simulink model "sscv_braking_ABS_w_vehicle"  (R2024a)
settings: Solver=ode23t  StartTime=0.0  StopTime=1  RelTol=1e-3  AbsTol=1e-3
PreLoadFcn:
  | sscv_braking_ABS_w_vehicle_input
values from neighbouring files (symbols this model uses):
  wheel_rad = 0.3    [sscv_braking_ABS_w_vehicle_input.m]
  wheel_vth = 0.01    [sscv_braking_ABS_w_vehicle_input.m]
undefined symbols (not defined in the file or in its folder): Asphalt, fcdb, HCU, MFormulaCoeff, tpc, vb
libraries: fl_lib x165, SimscapeFluids_lib x24, nesl_utility x21, sdl_lib x9, simulink x3, simulink_extras x1
(part 2 of 6)

== system sscv_braking_ABS_w_vehicle/Brakes with ABS/FCDB/RLW ==
  CP1 : fl_lib/Isothermal Liquid/Elements/Translational Mechanical Converter (IL)  mech_orientation=1  displacement_spec=foundation.enum.DisplacementSpec.Calculate  x0=0 m  interface_area=fcdb.area m^2  dead_volume=fcdb.deadV m^3  pressure_spec=1  environment_pressure=0.101325 MPa  dynamic_compressibility=simscape.enum.onoff.on  p0=tpc.pRes Pa
      settings: InternalSimscapePortConfiguration="{\"Bottom\":[],\"Left\":[{\"id\":\"A\",\"label\":\"A\",\"type\":\"foundation.isothermal_liquid.isothermal_liquid\"},{\"id\":\"C\",\"label\":\"C\",\"type\":\"foundation.mechanical.translational.translational\"}],\"Right\":[{\"id\":\"R\",\"label\":\"R\",\"type\":\"foundation.mechanical.translational.translational\"}],\"Top\":[]}"
  CP2 : fl_lib/Isothermal Liquid/Elements/Translational Mechanical Converter (IL)  mech_orientation=1  displacement_spec=foundation.enum.DisplacementSpec.Calculate  x0=0 m  interface_area=fcdb.area m^2  dead_volume=fcdb.deadV m^3  pressure_spec=1  environment_pressure=0.101325 MPa  dynamic_compressibility=simscape.enum.onoff.on  p0=tpc.pRes Pa
      settings: InternalSimscapePortConfiguration="{\"Bottom\":[],\"Left\":[{\"id\":\"A\",\"label\":\"A\",\"type\":\"foundation.isothermal_liquid.isothermal_liquid\"},{\"id\":\"C\",\"label\":\"C\",\"type\":\"foundation.mechanical.translational.translational\"}],\"Right\":[{\"id\":\"R\",\"label\":\"R\",\"type\":\"foundation.mechanical.translational.translational\"}],\"Top\":[]}"
  Ideal Force Sensor : fl_lib/Mechanical/Mechanical Sensors/Ideal Force Sensor
  Ideal Force Sensor1 : fl_lib/Mechanical/Mechanical Sensors/Ideal Force Sensor
  Loaded-Contact Rotational Friction : sdl_lib/Brakes & Detents/Rotational/Loaded-Contact Rotational Friction  geometry_model=sdl.enum.friction_geometry.radius  r_eff=fcdb.reffR m  d_o=150 mm  d_i=100 mm  enable_faults=simscape.enum.onoff.off  fault_type=sdl.enum.clutchFault.lock  friction_model=sdl.enum.friction_model_TLU_thermal.fixed  mu_w_vector=[0, 100, 1000] rad/s  temperature_TLU=[280, 300, 320] K  mu_static=fcdb.statFric  mu_static_vector=[.4, .38, .36]  mu_coulomb=fcdb.kinFric  mu_coulomb_vector=[.3, .22, .19]  mu_coulomb_temp_vector=[.3, .28, .25]  mu_coulomb_matrix=[.34, .32, .3; .3, .28, .25; .25, .2, .15]  mu_interp_method=simscape.enum.interpolation.linear  mu_extrap_method=simscape.enum.extrapolation.linear  w_tol=0.01 rad/s  force_min=1 N  mu_visc=fcdb.dampDisk N*m/(rad/s)  initial_state_locked=sdl.enum.initial_lock.unlocked  thermal_mass=50 kJ/K  T_init=300 K
      settings: InternalSimscapePortConfiguration="{\"Bottom\":[],\"Left\":[{\"id\":\"N\",\"label\":\"N\",\"type\":\"input\"},{\"id\":\"B\",\"label\":\"B\",\"type\":\"foundation.mechanical.rotational.rotational\"}],\"Right\":[{\"id\":\"F\",\"label\":\"F\",\"type\":\"foundation.mechanical.rotational.rotational\"}],\"Top\":[]}"
  Mass : fl_lib/Mechanical/Translational Elements/Mass  mass=fcdb.mass kg  num_ports=foundation.enum.numPorts2.one  v_specify=off  v_priority=High  v=0 m/s  v_nominal_specify=off  v_nominal_value=1  v_nominal_unit=m/s  f_specify=off  f_priority=None  f=0 N  f_nominal_specify=off  f_nominal_value=1  f_nominal_unit=N
  Mass1 : fl_lib/Mechanical/Translational Elements/Mass  mass=fcdb.mass kg  num_ports=foundation.enum.numPorts2.one  v_specify=off  v_priority=High  v=0 m/s  v_nominal_specify=off  v_nominal_value=1  v_nominal_unit=m/s  f_specify=off  f_priority=None  f=0 N  f_nominal_specify=off  f_nominal_value=1  f_nominal_unit=N
  Mechanical Rotational Reference : fl_lib/Mechanical/Rotational Elements/Mechanical Rotational Reference
  Mechanical Translational Reference : fl_lib/Mechanical/Translational Elements/Mechanical Translational Reference
  PS Add : fl_lib/Physical Signals/Functions/PS Add
  Translational Damper : fl_lib/Mechanical/Translational Elements/Translational Damper  D=fcdb.damp N/(m/s)  v_specify=off  v_priority=None  v=0 m/s  v_nominal_specify=off  v_nominal_value=1  v_nominal_unit=m/s  f_specify=off  f_priority=None  f=0 N  f_nominal_specify=off  f_nominal_value=1  f_nominal_unit=N
  Translational Damper1 : fl_lib/Mechanical/Translational Elements/Translational Damper  D=fcdb.damp N/(m/s)  v_specify=off  v_priority=None  v=0 m/s  v_nominal_specify=off  v_nominal_value=1  v_nominal_unit=m/s  f_specify=off  f_priority=None  f=0 N  f_nominal_specify=off  f_nominal_value=1  f_nominal_unit=N
  Translational Hard Stop : fl_lib/Mechanical/Translational Elements/Translational Hard Stop  upper_bnd=fcdb.runClear m  lower_bnd=0 m  model=simscape.enum.hardstop.smooth  stiff_up=fcdb.complianceR N/m  stiff_low=fcdb.hss N/m  D_up=fcdb.damp N/(m/s)  D_low=fcdb.hsd N/(m/s)  transition=0.1 mm  coeff_rest=0.7  v_tol=0.001 m/s  f_tol=0.001 N  v_specify=off  v_priority=None  v=0 m/s  v_nominal_specify=off  v_nominal_value=1  v_nominal_unit=m/s  f_specify=off  f_priority=None  f=0 N  f_nominal_specify=off  f_nominal_value=1  f_nominal_unit=N  x_specify=off  x_priority=High  x=0 m  x_nominal_specify=off  x_nominal_value=1  x_nominal_unit=m  M_specify=off  M_priority=None  M=0
  Translational Hard Stop1 : fl_lib/Mechanical/Translational Elements/Translational Hard Stop  upper_bnd=fcdb.runClear m  lower_bnd=0 m  model=simscape.enum.hardstop.smooth  stiff_up=fcdb.complianceR N/m  stiff_low=fcdb.hss N/m  D_up=fcdb.damp N/(m/s)  D_low=fcdb.hsd N/(m/s)  transition=0.1 mm  coeff_rest=0.7  v_tol=0.001 m/s  f_tol=0.001 N  v_specify=off  v_priority=None  v=0 m/s  v_nominal_specify=off  v_nominal_value=1  v_nominal_unit=m/s  f_specify=off  f_priority=None  f=0 N  f_nominal_specify=off  f_nominal_value=1  f_nominal_unit=N  x_specify=off  x_priority=High  x=0 m  x_nominal_specify=off  x_nominal_value=1  x_nominal_unit=m  M_specify=off  M_priority=None  M=0
  Brk2 : PMIOPort  Side=Left
  TRLW : PMIOPort  Port=2  Side=Right
  connections:
  Ideal Force Sensor/LConn1 -- Translational Damper/RConn1 -- Translational Hard Stop/RConn1
  Ideal Force Sensor/RConn1 -- CP1/LConn2 -- CP2/LConn2 -- Ideal Force Sensor1/RConn1 -- Mechanical Translational Reference/LConn1
  Translational Damper1/LConn1 -- CP2/RConn1 -- Mass1/LConn1 -- Translational Hard Stop1/LConn1
  Ideal Force Sensor1/LConn1 -- Translational Damper1/RConn1 -- Translational Hard Stop1/RConn1
  PS Add/LConn1 -- Ideal Force Sensor/RConn2
  Ideal Force Sensor1/RConn2 -- PS Add/LConn2
  PS Add/RConn1 -- Loaded-Contact Rotational Friction/LConn1
  Mechanical Rotational Reference/LConn1 -- Loaded-Contact Rotational Friction/LConn2
  TRLW/RConn1 -- Loaded-Contact Rotational Friction/RConn1
  Brk2/RConn1 -- CP2/LConn1 -- CP1/LConn1
  Translational Damper/LConn1 -- Mass/LConn1 -- CP1/RConn1 -- Translational Hard Stop/LConn1

== system sscv_braking_ABS_w_vehicle/Brakes with ABS/FCDB/RRW ==
  CP1 : fl_lib/Isothermal Liquid/Elements/Translational Mechanical Converter (IL)  mech_orientation=1  displacement_spec=foundation.enum.DisplacementSpec.Calculate  x0=0 m  interface_area=fcdb.area m^2  dead_volume=fcdb.deadV m^3  pressure_spec=1  environment_pressure=0.101325 MPa  dynamic_compressibility=simscape.enum.onoff.on  p0=tpc.pRes Pa
      settings: InternalSimscapePortConfiguration="{\"Bottom\":[],\"Left\":[{\"id\":\"A\",\"label\":\"A\",\"type\":\"foundation.isothermal_liquid.isothermal_liquid\"},{\"id\":\"C\",\"label\":\"C\",\"type\":\"foundation.mechanical.translational.translational\"}],\"Right\":[{\"id\":\"R\",\"label\":\"R\",\"type\":\"foundation.mechanical.translational.translational\"}],\"Top\":[]}"
  CP2 : fl_lib/Isothermal Liquid/Elements/Translational Mechanical Converter (IL)  mech_orientation=1  displacement_spec=foundation.enum.DisplacementSpec.Calculate  x0=0 m  interface_area=fcdb.area m^2  dead_volume=fcdb.deadV m^3  pressure_spec=1  environment_pressure=0.101325 MPa  dynamic_compressibility=simscape.enum.onoff.on  p0=tpc.pRes Pa
      settings: InternalSimscapePortConfiguration="{\"Bottom\":[],\"Left\":[{\"id\":\"A\",\"label\":\"A\",\"type\":\"foundation.isothermal_liquid.isothermal_liquid\"},{\"id\":\"C\",\"label\":\"C\",\"type\":\"foundation.mechanical.translational.translational\"}],\"Right\":[{\"id\":\"R\",\"label\":\"R\",\"type\":\"foundation.mechanical.translational.translational\"}],\"Top\":[]}"
  Ideal Force Sensor : fl_lib/Mechanical/Mechanical Sensors/Ideal Force Sensor
  Ideal Force Sensor1 : fl_lib/Mechanical/Mechanical Sensors/Ideal Force Sensor
  Loaded-Contact Rotational Friction : sdl_lib/Brakes & Detents/Rotational/Loaded-Contact Rotational Friction  geometry_model=sdl.enum.friction_geometry.radius  r_eff=fcdb.reffR m  d_o=150 mm  d_i=100 mm  enable_faults=simscape.enum.onoff.off  fault_type=sdl.enum.clutchFault.lock  friction_model=sdl.enum.friction_model_TLU_thermal.fixed  mu_w_vector=[0, 100, 1000] rad/s  temperature_TLU=[280, 300, 320] K  mu_static=fcdb.statFric  mu_static_vector=[.4, .38, .36]  mu_coulomb=fcdb.kinFric  mu_coulomb_vector=[.3, .22, .19]  mu_coulomb_temp_vector=[.3, .28, .25]  mu_coulomb_matrix=[.34, .32, .3; .3, .28, .25; .25, .2, .15]  mu_interp_method=simscape.enum.interpolation.linear  mu_extrap_method=simscape.enum.extrapolation.linear  w_tol=0.01 rad/s  force_min=1 N  mu_visc=fcdb.dampDisk N*m/(rad/s)  initial_state_locked=sdl.enum.initial_lock.unlocked  thermal_mass=50 kJ/K  T_init=300 K
      settings: InternalSimscapePortConfiguration="{\"Bottom\":[],\"Left\":[{\"id\":\"N\",\"label\":\"N\",\"type\":\"input\"},{\"id\":\"B\",\"label\":\"B\",\"type\":\"foundation.mechanical.rotational.rotational\"}],\"Right\":[{\"id\":\"F\",\"label\":\"F\",\"type\":\"foundation.mechanical.rotational.rotational\"}],\"Top\":[]}"
  Mass : fl_lib/Mechanical/Translational Elements/Mass  mass=fcdb.mass kg  num_ports=foundation.enum.numPorts2.one  v_specify=off  v_priority=High  v=0 m/s  v_nominal_specify=off  v_nominal_value=1  v_nominal_unit=m/s  f_specify=off  f_priority=None  f=0 N  f_nominal_specify=off  f_nominal_value=1  f_nominal_unit=N
  Mass1 : fl_lib/Mechanical/Translational Elements/Mass  mass=fcdb.mass kg  num_ports=foundation.enum.numPorts2.one  v_specify=off  v_priority=High  v=0 m/s  v_nominal_specify=off  v_nominal_value=1  v_nominal_unit=m/s  f_specify=off  f_priority=None  f=0 N  f_nominal_specify=off  f_nominal_value=1  f_nominal_unit=N
  Mechanical Rotational Reference : fl_lib/Mechanical/Rotational Elements/Mechanical Rotational Reference
  Mechanical Translational Reference : fl_lib/Mechanical/Translational Elements/Mechanical Translational Reference
  PS Add : fl_lib/Physical Signals/Functions/PS Add
  Translational Damper : fl_lib/Mechanical/Translational Elements/Translational Damper  D=fcdb.damp N/(m/s)  v_specify=off  v_priority=None  v=0 m/s  v_nominal_specify=off  v_nominal_value=1  v_nominal_unit=m/s  f_specify=off  f_priority=None  f=0 N  f_nominal_specify=off  f_nominal_value=1  f_nominal_unit=N
  Translational Damper1 : fl_lib/Mechanical/Translational Elements/Translational Damper  D=fcdb.damp N/(m/s)  v_specify=off  v_priority=None  v=0 m/s  v_nominal_specify=off  v_nominal_value=1  v_nominal_unit=m/s  f_specify=off  f_priority=None  f=0 N  f_nominal_specify=off  f_nominal_value=1  f_nominal_unit=N
  Translational Hard Stop : fl_lib/Mechanical/Translational Elements/Translational Hard Stop  upper_bnd=fcdb.runClear m  lower_bnd=0 m  model=simscape.enum.hardstop.smooth  stiff_up=fcdb.complianceR N/m  stiff_low=fcdb.hss N/m  D_up=fcdb.damp N/(m/s)  D_low=fcdb.hsd N/(m/s)  transition=0.1 mm  coeff_rest=0.7  v_tol=0.001 m/s  f_tol=0.001 N  v_specify=off  v_priority=None  v=0 m/s  v_nominal_specify=off  v_nominal_value=1  v_nominal_unit=m/s  f_specify=off  f_priority=None  f=0 N  f_nominal_specify=off  f_nominal_value=1  f_nominal_unit=N  x_specify=off  x_priority=High  x=0 m  x_nominal_specify=off  x_nominal_value=1  x_nominal_unit=m  M_specify=off  M_priority=None  M=0
  Translational Hard Stop1 : fl_lib/Mechanical/Translational Elements/Translational Hard Stop  upper_bnd=fcdb.runClear m  lower_bnd=0 m  model=simscape.enum.hardstop.smooth  stiff_up=fcdb.complianceR N/m  stiff_low=fcdb.hss N/m  D_up=fcdb.damp N/(m/s)  D_low=fcdb.hsd N/(m/s)  transition=0.1 mm  coeff_rest=0.7  v_tol=0.001 m/s  f_tol=0.001 N  v_specify=off  v_priority=None  v=0 m/s  v_nominal_specify=off  v_nominal_value=1  v_nominal_unit=m/s  f_specify=off  f_priority=None  f=0 N  f_nominal_specify=off  f_nominal_value=1  f_nominal_unit=N  x_specify=off  x_priority=High  x=0 m  x_nominal_specify=off  x_nominal_value=1  x_nominal_unit=m  M_specify=off  M_priority=None  M=0
  Brk2 : PMIOPort  Side=Left
  TRRW : PMIOPort  Port=2  Side=Right
  connections:
  Ideal Force Sensor1/RConn2 -- PS Add/LConn2
  PS Add/LConn1 -- Ideal Force Sensor/RConn2
  Translational Damper1/RConn1 -- Translational Hard Stop1/RConn1 -- Ideal Force Sensor1/LConn1
  Mechanical Translational Reference/LConn1 -- Ideal Force Sensor1/RConn1 -- CP2/LConn2 -- Ideal Force Sensor/RConn1 -- CP1/LConn2
  Translational Hard Stop/RConn1 -- Translational Damper/RConn1 -- Ideal Force Sensor/LConn1
  PS Add/RConn1 -- Loaded-Contact Rotational Friction/LConn1
  Mechanical Rotational Reference/LConn1 -- Loaded-Contact Rotational Friction/LConn2
  TRRW/RConn1 -- Loaded-Contact Rotational Friction/RConn1
  Mass/LConn1 -- Translational Hard Stop/LConn1 -- Translational Damper/LConn1 -- CP1/RConn1
  Brk2/RConn1 -- CP2/LConn1 -- CP1/LConn1
  Translational Hard Stop1/LConn1 -- Mass1/LConn1 -- CP2/RConn1 -- Translational Damper1/LConn1

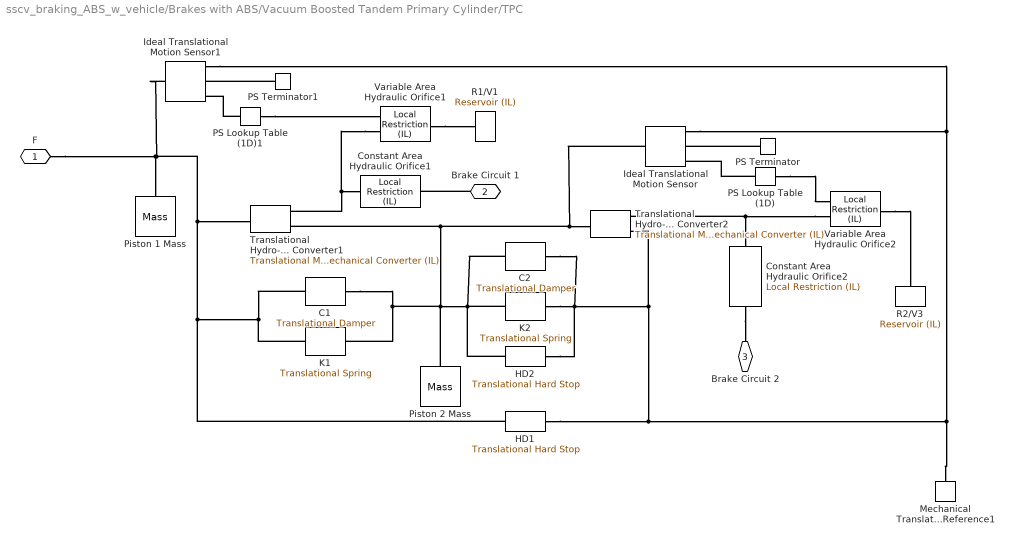
== system sscv_braking_ABS_w_vehicle/Brakes with ABS/Vacuum Boosted Tandem Primary Cylinder/TPC ==
  C1 : fl_lib/Mechanical/Translational Elements/Translational Damper  D=tpc.c1 N/(m/s)  v_specify=off  v_priority=None  v=0 m/s  v_nominal_specify=off  v_nominal_value=1  v_nominal_unit=m/s  f_specify=off  f_priority=None  f=0 N  f_nominal_specify=off  f_nominal_value=1  f_nominal_unit=N
  C2 : fl_lib/Mechanical/Translational Elements/Translational Damper  D=tpc.c2 N/(m/s)  v_specify=off  v_priority=None  v=0 m/s  v_nominal_specify=off  v_nominal_value=1  v_nominal_unit=m/s  f_specify=off  f_priority=None  f=0 N  f_nominal_specify=off  f_nominal_value=1  f_nominal_unit=N
  Constant Area Hydraulic Orifice1 : fl_lib/Isothermal Liquid/Elements/Local Restriction (IL)  restriction_type=1  restriction_area=tpc.a2Ori m^2  min_area=1e-10 m^2  max_area=0.005 m^2  area=inf m^2  Cd=0.7  Re_c=150  pressure_recovery=simscape.enum.onoff.off
      settings: InternalSimscapePortConfiguration="{\"Bottom\":[],\"Left\":[{\"id\":\"A\",\"label\":\"A\",\"type\":\"foundation.isothermal_liquid.isothermal_liquid\"}],\"Right\":[{\"id\":\"B\",\"label\":\"B\",\"type\":\"foundation.isothermal_liquid.isothermal_liquid\"}],\"Top\":[]}"
  Constant Area Hydraulic Orifice2 : fl_lib/Isothermal Liquid/Elements/Local Restriction (IL)  restriction_type=1  restriction_area=tpc.a2Ori m^2  min_area=1e-10 m^2  max_area=0.005 m^2  area=inf m^2  Cd=0.7  Re_c=150  pressure_recovery=simscape.enum.onoff.off
      settings: InternalSimscapePortConfiguration="{\"Bottom\":[],\"Left\":[{\"id\":\"A\",\"label\":\"A\",\"type\":\"foundation.isothermal_liquid.isothermal_liquid\"}],\"Right\":[{\"id\":\"B\",\"label\":\"B\",\"type\":\"foundation.isothermal_liquid.isothermal_liquid\"}],\"Top\":[]}"
  HD1 : fl_lib/Mechanical/Translational Elements/Translational Hard Stop  upper_bnd=tpc.x13 m  lower_bnd=0 m  model=simscape.enum.hardstop.smooth  stiff_up=tpc.hss N/m  stiff_low=tpc.hss N/m  D_up=tpc.hsd N/(m/s)  D_low=tpc.hsd N/(m/s)  transition=0.1 mm  coeff_rest=0.7  v_tol=0.001 m/s  f_tol=0.001 N  v_specify=off  v_priority=None  v=0 m/s  v_nominal_specify=off  v_nominal_value=1  v_nominal_unit=m/s  f_specify=off  f_priority=None  f=0 N  f_nominal_specify=off  f_nominal_value=1  f_nominal_unit=N  x_specify=off  x_priority=High  x=0 m  x_nominal_specify=off  x_nominal_value=1  x_nominal_unit=m  M_specify=off  M_priority=None  M=0
  HD2 : fl_lib/Mechanical/Translational Elements/Translational Hard Stop  upper_bnd=tpc.x23 m  lower_bnd=0 m  model=simscape.enum.hardstop.smooth  stiff_up=tpc.hss N/m  stiff_low=tpc.hss N/m  D_up=tpc.hsd N/(m/s)  D_low=tpc.hsd N/(m/s)  transition=0.1 mm  coeff_rest=0.7  v_tol=0.001 m/s  f_tol=0.001 N  v_specify=off  v_priority=None  v=0 m/s  v_nominal_specify=off  v_nominal_value=1  v_nominal_unit=m/s  f_specify=off  f_priority=None  f=0 N  f_nominal_specify=off  f_nominal_value=1  f_nominal_unit=N  x_specify=off  x_priority=High  x=0 m  x_nominal_specify=off  x_nominal_value=1  x_nominal_unit=m  M_specify=off  M_priority=None  M=0
  Ideal Translational Motion Sensor : fl_lib/Mechanical/Mechanical Sensors/Ideal Translational Motion Sensor  reference=foundation.enum.MeasurementReference.difference  acceleration_port=false  velocity_port=true  position_port=true  offset=0 m
  Ideal Translational Motion Sensor1 : fl_lib/Mechanical/Mechanical Sensors/Ideal Translational Motion Sensor  reference=foundation.enum.MeasurementReference.difference  acceleration_port=false  velocity_port=true  position_port=true  offset=0 m
  K1 : fl_lib/Mechanical/Translational Elements/Translational Spring  spr_rate=tpc.k1 N/m  v_specify=off  v_priority=None  v=0 m/s  v_nominal_specify=off  v_nominal_value=1  v_nominal_unit=m/s  f_specify=off  f_priority=None  f=0 N  f_nominal_specify=off  f_nominal_value=1  f_nominal_unit=N  x_specify=on  x_priority=High  x=tpc.defLL m  x_nominal_specify=off  x_nominal_value=1  x_nominal_unit=m
  K2 : fl_lib/Mechanical/Translational Elements/Translational Spring  spr_rate=tpc.k2 N/m  v_specify=off  v_priority=None  v=0 m/s  v_nominal_specify=off  v_nominal_value=1  v_nominal_unit=m/s  f_specify=off  f_priority=None  f=0 N  f_nominal_specify=off  f_nominal_value=1  f_nominal_unit=N  x_specify=on  x_priority=High  x=tpc.defLR m  x_nominal_specify=off  x_nominal_value=1  x_nominal_unit=m
  Mechanical Translational Reference1 : fl_lib/Mechanical/Translational Elements/Mechanical Translational Reference
  PS Lookup Table (1D) : fl_lib/Physical Signals/Lookup Tables/PS Lookup Table (1D)  x=[0 tpc.x22 tpc.x23] m  f=[tpc.a1Ori 0 0] m^2  interp_method=simscape.enum.interpolation.linear  extrap_method=simscape.enum.extrapolation.linear
  PS Lookup Table (1D)1 : fl_lib/Physical Signals/Lookup Tables/PS Lookup Table (1D)  x=[0 tpc.x12 tpc.x13] m  f=[tpc.a1Ori 0 0] m^2  interp_method=simscape.enum.interpolation.linear  extrap_method=simscape.enum.extrapolation.linear
  PS Terminator : fl_lib/Physical Signals/Sinks/PS Terminator
  PS Terminator1 : fl_lib/Physical Signals/Sinks/PS Terminator
  Piston 1 Mass : fl_lib/Mechanical/Translational Elements/Mass  mass=tpc.mass1 kg  num_ports=foundation.enum.numPorts2.one  v_specify=off  v_priority=High  v=0 m/s  v_nominal_specify=off  v_nominal_value=1  v_nominal_unit=m/s  f_specify=off  f_priority=None  f=0 N  f_nominal_specify=off  f_nominal_value=1  f_nominal_unit=N
  Piston 2 Mass : fl_lib/Mechanical/Translational Elements/Mass  mass=tpc.mass2 kg  num_ports=foundation.enum.numPorts2.one  v_specify=off  v_priority=High  v=0 m/s  v_nominal_specify=off  v_nominal_value=1  v_nominal_unit=m/s  f_specify=off  f_priority=None  f=0 N  f_nominal_specify=off  f_nominal_value=1  f_nominal_unit=N
  R1/V1 : fl_lib/Isothermal Liquid/Elements/Reservoir (IL)  reservoir_type=foundation.enum.constant_controlled.constant  pressure_spec=foundation.enum.pressure_spec.atmospheric  reservoir_pressure=0.101325 MPa
  R2/V3 : fl_lib/Isothermal Liquid/Elements/Reservoir (IL)  reservoir_type=foundation.enum.constant_controlled.constant  pressure_spec=foundation.enum.pressure_spec.atmospheric  reservoir_pressure=0.101325 MPa
  Translational Hydro-Mechanical Converter1 : fl_lib/Isothermal Liquid/Elements/Translational Mechanical Converter (IL)  mech_orientation=-1  displacement_spec=foundation.enum.DisplacementSpec.Calculate  x0=-(tpc.x13-tpc.x23) m  interface_area=tpc.aPist m^2  dead_volume=tpc.v2D m^3  pressure_spec=1  environment_pressure=0.101325 MPa  dynamic_compressibility=simscape.enum.onoff.on  p0=tpc.pRes Pa
      settings: InternalSimscapePortConfiguration="{\"Bottom\":[],\"Left\":[{\"id\":\"A\",\"label\":\"A\",\"type\":\"foundation.isothermal_liquid.isothermal_liquid\"},{\"id\":\"C\",\"label\":\"C\",\"type\":\"foundation.mechanical.translational.translational\"}],\"Right\":[{\"id\":\"R\",\"label\":\"R\",\"type\":\"foundation.mechanical.translational.translational\"}],\"Top\":[]}"
  Translational Hydro-Mechanical Converter2 : fl_lib/Isothermal Liquid/Elements/Translational Mechanical Converter (IL)  mech_orientation=-1  displacement_spec=foundation.enum.DisplacementSpec.Calculate  x0=-(tpc.x23) m  interface_area=tpc.aPist m^2  dead_volume=tpc.v4D m^3  pressure_spec=1  environment_pressure=0.101325 MPa  dynamic_compressibility=simscape.enum.onoff.on  p0=tpc.pRes Pa
      settings: InternalSimscapePortConfiguration="{\"Bottom\":[],\"Left\":[{\"id\":\"A\",\"label\":\"A\",\"type\":\"foundation.isothermal_liquid.isothermal_liquid\"},{\"id\":\"C\",\"label\":\"C\",\"type\":\"foundation.mechanical.translational.translational\"}],\"Right\":[{\"id\":\"R\",\"label\":\"R\",\"type\":\"foundation.mechanical.translational.translational\"}],\"Top\":[]}"
  Variable Area Hydraulic Orifice1 : fl_lib/Isothermal Liquid/Elements/Local Restriction (IL)  restriction_type=foundation.enum.restriction_type.variable  restriction_area=1e-3 m^2  min_area=1e-12 m^2  max_area=1e10 m^2  area=inf m^2  Cd=0.7  Re_c=150  pressure_recovery=simscape.enum.onoff.off
      settings: InternalSimscapePortConfiguration="{\"Bottom\":[],\"Left\":[{\"id\":\"A\",\"label\":\"A\",\"type\":\"foundation.isothermal_liquid.isothermal_liquid\"},{\"id\":\"AR\",\"label\":\"AR\",\"type\":\"input\"}],\"Right\":[{\"id\":\"B\",\"label\":\"B\",\"type\":\"foundation.isothermal_liquid.isothermal_liquid\"}],\"Top\":[]}"
  Variable Area Hydraulic Orifice2 : fl_lib/Isothermal Liquid/Elements/Local Restriction (IL)  restriction_type=foundation.enum.restriction_type.variable  restriction_area=1e-3 m^2  min_area=1e-12 m^2  max_area=1e10 m^2  area=inf m^2  Cd=0.7  Re_c=150  pressure_recovery=simscape.enum.onoff.off
      settings: InternalSimscapePortConfiguration="{\"Bottom\":[],\"Left\":[{\"id\":\"A\",\"label\":\"A\",\"type\":\"foundation.isothermal_liquid.isothermal_liquid\"},{\"id\":\"AR\",\"label\":\"AR\",\"type\":\"input\"}],\"Right\":[{\"id\":\"B\",\"label\":\"B\",\"type\":\"foundation.isothermal_liquid.isothermal_liquid\"}],\"Top\":[]}"
  F : PMIOPort  Side=Right
  Brake Circuit 1 : PMIOPort  Port=2  Side=Left
  Brake Circuit 2 : PMIOPort  Port=3  Side=Left
  connections:
  PS Terminator1/LConn1 -- Ideal Translational Motion Sensor1/RConn2
  PS Terminator/LConn1 -- Ideal Translational Motion Sensor/RConn2
  PS Lookup Table (1D)/LConn1 -- Ideal Translational Motion Sensor/RConn3
  PS Lookup Table (1D)1/LConn1 -- Ideal Translational Motion Sensor1/RConn3
  Constant Area Hydraulic Orifice2/RConn1 -- Brake Circuit 2/RConn1
  Variable Area Hydraulic Orifice1/RConn1 -- R1/V1/LConn1
  Variable Area Hydraulic Orifice2/RConn1 -- R2/V3/LConn1
  PS Lookup Table (1D)1/RConn1 -- Variable Area Hydraulic Orifice1/LConn2
  Brake Circuit 1/RConn1 -- Constant Area Hydraulic Orifice1/RConn1
  Variable Area Hydraulic Orifice1/LConn1 -- Translational Hydro-Mechanical Converter1/LConn1 -- Constant Area Hydraulic Orifice1/LConn1
  HD1/LConn1 -- C1/LConn1 -- K1/LConn1 -- Translational Hydro-Mechanical Converter1/RConn1 -- F/RConn1 -- Piston 1 Mass/LConn1 -- Ideal Translational Motion Sensor1/LConn1
  PS Lookup Table (1D)/RConn1 -- Variable Area Hydraulic Orifice2/LConn2
  C1/RConn1 -- Translational Hydro-Mechanical Converter1/LConn2 -- Ideal Translational Motion Sensor/LConn1 -- Translational Hydro-Mechanical Converter2/RConn1 -- C2/LConn1 -- HD2/LConn1 -- K2/LConn1 -- Piston 2 Mass/LConn1 -- K1/RConn1
  Ideal Translational Motion Sensor1/RConn1 -- Ideal Translational Motion Sensor/RConn1 -- Mechanical Translational Reference1/LConn1 -- HD2/RConn1 -- C2/RConn1 -- K2/RConn1 -- Translational Hydro-Mechanical Converter2/LConn2 -- HD1/RConn1
  Variable Area Hydraulic Orifice2/LConn1 -- Translational Hydro-Mechanical Converter2/LConn1 -- Constant Area Hydraulic Orifice2/LConn1
